simulink model "both_MPC_off_grid"  (R2015b)
settings: Solver=ode5  StartTime=0.0  StopTime=5  RelTol=1e-3
libraries: powerlib x27, powerlib_meascontrol x6, powerlib_extras x1
settings Model: Creator=fujitsu  LastModifiedBy=fujitsu

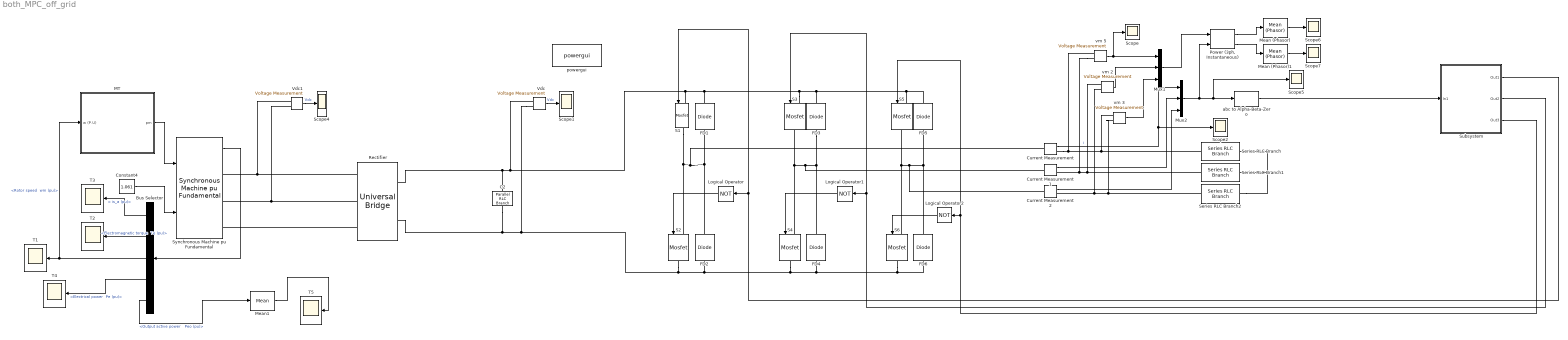
== system both_MPC_off_grid ==
  Bus Selector : BusSelector  OutputSignals="Stator current. is_a (pu),Mechanical.Electromagnetic torque  Te (pu),Mechanical.Rotor speed  wm (pu),Mechanical.Electrical power  Pe (pu),Output active power   Peo (pu)"
  C2 : powerlib/Elements/Parallel RLC Branch  LConnTagsString=a  RConnTagsString=__new0  BranchType=C  Resistance=inf  Inductance=inf  SetiL0=off  InitialCurrent=0  Capacitance=5000e-06  Setx0=off  InitialVoltage=0  Measurements=None
  Constant4 : Constant  Value=1.061
  Current Measurement : powerlib/Measurements/Current Measurement  PhasorSimulation=off  OutputType=Complex  PSBequivalent=0
  Current Measurement1 : powerlib/Measurements/Current Measurement  PhasorSimulation=off  OutputType=Complex  PSBequivalent=0
  Current Measurement2 : powerlib/Measurements/Current Measurement  PhasorSimulation=off  OutputType=Complex  PSBequivalent=0
  FD{1..6} (6 alike) : powerlib/Power Electronics/Diode  Ron=0.001  Lon=0  Vf=0.8  IC=0  UseSnubber=off  Rs=500  Cs=250e-9  Measurements=off
  Logical Operator : Logic  Operator=NOT  AllPortsSameDT=off  OutDataTypeStr=boolean
  Logical Operator1 : Logic  Operator=NOT  AllPortsSameDT=off  OutDataTypeStr=boolean
  Logical Operator2 : Logic  Operator=NOT  AllPortsSameDT=off  OutDataTypeStr=boolean
  MT : Subsystem
  Mean (Phasor) : powerlib_meascontrol/Measurements/Mean (Phasor)  Freq=50  Vinit=0  Ts=0
  Mean (Phasor)1 : powerlib_meascontrol/Measurements/Mean (Phasor)  Freq=50  Vinit=0  Ts=0
  Mean1 : powerlib_meascontrol/Measurements/Mean  Freq=50  Vinit=0  Ts=1e-6
  Mux1 : Mux  Inputs=3
  Mux2 : Mux  Inputs=3
  "Power (3ph, Instantaneous)" : powerlib_meascontrol/Measurements/Power (3ph, Instantaneous)
  Rectifier : powerlib/Power Electronics/Universal Bridge  Arms=3  SnubberResistance=50  SnubberCapacitance=0.1e-6  Device=Diodes  Ron=1e-3  Lon=0  ForwardVoltages="[  0.8  0.8  ]"  ForwardVoltage=.7  GTOparameters=[ 10e-6 , 20e-6 ]  IGBTparameters=[ 1e-6 , 2e-6 ]  Measurements=Device currents  Measurements_2=None  converterType=Rectifier
  S{1..6} (6 alike) : powerlib/Power Electronics/Mosfet  Ron=0.1  Lon=0  Rd=0.01  Vfd=0  IC=0  Rs=1e5  Cs=inf  Measurements=off
  Scope{,1..2,4..7} (7 alike) : Scope
  Series RLC Branch : powerlib/Elements/Series RLC Branch  LConnTagsString=__new0  RConnTagsString=__new0  BranchType=RL  Resistance=765^2/50000  Inductance=10e-3  SetiL0=off  InitialCurrent=0  Capacitance=1e-6  Setx0=off  InitialVoltage=0  Measurements=None
  Series RLC Branch1 : powerlib/Elements/Series RLC Branch  LConnTagsString=__new0  RConnTagsString=__new0  BranchType=RL  Resistance=765^2/50000  Inductance=10e-3  SetiL0=off  InitialCurrent=0  Capacitance=1e-6  Setx0=off  InitialVoltage=0  Measurements=None
  Series RLC Branch2 : powerlib/Elements/Series RLC Branch  LConnTagsString=__new0  RConnTagsString=__new0  BranchType=RL  Resistance=765^2/50000  Inductance=10e-3  SetiL0=off  InitialCurrent=0  Capacitance=1e-6  Setx0=off  InitialVoltage=0  Measurements=None
  Subsystem : Subsystem
  Synchronous Machine pu Fundamental : powerlib/Machines/Synchronous Machine pu Fundamental  PresetModel=No  MechanicalLoad=Mechanical power Pm  ShowDetailedParameters=on  RotorType=Salient-pole  Units=per unit fundamental parameters  MeasurementBus=off  NominalParameters="[ 65e3  580 1600]"  Stator="[ 0.2503  0.114  0.6875  0.6875 ]"  Field="[ 1  10e15/(100*pi)]"  Dampers2=[0.0652, 0.5134, 0.0287, 0.2553, 7.765e-3, 0.9167 ]  Dampers1="[ 1.17E-02  0.182  1.97E-02  0.384 ]"  Mechanical=[ 6 0 2]  PolePairs=20  InitialConditions="[ 0  0  0  0  0  0  0  0  1 ]"  SetSaturation=off  Saturation=[0.6404,0.7127,0.8441,0.9214,0.9956,1.082,1.19,1.316,1.457;0.7,0.7698,0.8872,0.9466,0.9969,1.046,1.1,1.151,1.201]  LoadFlowParameters=[1,0,0,0,0]  TsPowergui=0  TsBlock=-1  IterativeModel=Trapezoidal non iterative  BusType=swing  Pref=0  Qref=0  Qmin=-inf  Qmax=inf  PLF=0  QLF=0
  T{1..5} (5 alike) : Scope
  Vdc : powerlib/Measurements/Voltage Measurement  Tag=PoWeRsYsTeMmEaSuReMeNt  PhasorSimulation=off  OutputType=Magnitude  PSBequivalent=0
  Vdc1 : powerlib/Measurements/Voltage Measurement  Tag=PoWeRsYsTeMmEaSuReMeNt  PhasorSimulation=off  OutputType=Magnitude  PSBequivalent=0
  abc to Alpha-Beta-Zero : powerlib_meascontrol/Transformations/abc to Alpha-Beta-Zero
  powergui : powerlib/powergui  SimulationMode=Continuous  SolverType=Tustin  SampleTime=5e-6  frequency=60  SPID=off  DisableSnubberDevices=off  DisableRonSwitches=off  DisableVfSwitches=off  SwTol=0  DisplayEquations=off  Interpol=off  ExternalGateDelay=off  methode=off  Ts=0  FunctionMessages=off  echomessages=off  HookPort=off  EnableUseOfTLC=off  x0status=blocks  frequencyindice=0  Pbase=100e6  ErrMax=0.0001  Iterations=50  UnitsV=kV  UnitsW=MW  buscounter=0  RestoreLinks=warning  ResistiveCurrentMeasurement=off  Frange=[0:2:500]  Ylog=off  Xlog=on  ShowGrid=off  save=off  variable=ZData  structure=ScopeData11111  ZoomFFT=off  StartTime=2  cycles=5  DisplayStyle=1  fundamental=50  FreqAxis=on  MaxFrequency=10000  frequencyindicesteady=1  RmsSteady=1  display=off
  vm 2 : powerlib/Measurements/Voltage Measurement  PhasorSimulation=off  OutputType=Complex  PSBequivalent=0
  vm 3 : powerlib/Measurements/Voltage Measurement  PhasorSimulation=off  OutputType=Complex  PSBequivalent=0
  vm 5 : powerlib/Measurements/Voltage Measurement  PhasorSimulation=off  OutputType=Complex  PSBequivalent=0
  wires:
  Vdc/1 -> Scope1/1  "Vdc"
  MT/1(pm) -> Synchronous Machine pu Fundamental/1
  Synchronous Machine pu Fundamental/1 -> Bus Selector/1
  Bus Selector/1 -> T3/1  "< is_a (pu)>"
  Bus Selector/2 -> T2/1  "<Electromagnetic torque  Te (pu)>"
  Bus Selector/3 -> MT/1(w (P.U)), T1/1  "<Rotor speed  wm (pu)>"
  Constant4/1 -> Synchronous Machine pu Fundamental/2
  Vdc1/1 -> Scope4/1  "Vdc"
  Bus Selector/4 -> T4/1  "<Electrical power  Pe (pu)>"
  Bus Selector/5 -> Mean1/1  "<Output active power   Peo (pu)>"
  Mean1/1 -> T5/1
  Current Measurement/1 -> Mux2/1, Scope2/1  "i"
  Current Measurement1/1 -> Mux2/2
  Current Measurement2/1 -> Mux2/3
  Mux2/1 -> "Power (3ph, Instantaneous)"/2, Scope5/1, abc to Alpha-Beta-Zero/1
  Logical Operator/1 -> S2/1
  Logical Operator1/1 -> S4/1
  Logical Operator2/1 -> S6/1
  vm 5/1 -> Scope/1, Mux1/1
  Subsystem/3(Out3) -> S5/1, Logical Operator2/1
  Subsystem/2(Out2) -> S3/1, Logical Operator1/1
  Subsystem/1(Out1) -> S1/1, Logical Operator/1
  abc to Alpha-Beta-Zero/1 -> Subsystem/1(In1)
  vm 2/1 -> Mux1/2
  vm 3/1 -> Mux1/3
  Mux1/1 -> "Power (3ph, Instantaneous)"/1
  "Power (3ph, Instantaneous)"/1 -> Mean (Phasor)/1
  "Power (3ph, Instantaneous)"/2 -> Mean (Phasor)1/1
  Mean (Phasor)/1 -> Scope6/1
  Mean (Phasor)1/1 -> Scope7/1
  connections:
  Current Measurement/RConn1 -- vm 5/LConn1 -- vm 3/LConn1 -- Series RLC Branch/LConn1
  S1/RConn1 -- S2/LConn1 -- Current Measurement/LConn1 -- FD1/LConn1 -- FD2/RConn1
  S3/RConn1 -- S4/LConn1 -- FD4/RConn1 -- FD3/LConn1 -- Current Measurement1/LConn1
  S5/RConn1 -- S6/LConn1 -- FD6/RConn1 -- FD5/LConn1 -- Current Measurement2/LConn1
  vm 5/LConn2 -- Current Measurement1/RConn1 -- Series RLC Branch1/LConn1 -- vm 2/LConn1
  Series RLC Branch1/RConn1 -- Series RLC Branch/RConn1 -- Series RLC Branch2/RConn1
  vm 2/LConn2 -- Current Measurement2/RConn1 -- Series RLC Branch2/LConn1 -- vm 3/LConn2
  Synchronous Machine pu Fundamental/RConn1 -- Vdc1/LConn1 -- Rectifier/LConn1
  Vdc/LConn2 -- Rectifier/RConn2 -- C2/RConn1 -- S2/RConn1 -- FD2/LConn1 -- S4/RConn1 -- S6/RConn1 -- FD6/LConn1 -- FD4/LConn1
  S3/LConn1 -- FD1/RConn1 -- Rectifier/RConn1 -- C2/LConn1 -- Vdc/LConn1 -- S1/LConn1 -- FD3/RConn1 -- FD5/RConn1 -- S5/LConn1
  Rectifier/LConn2 -- Vdc1/LConn2 -- Synchronous Machine pu Fundamental/RConn2
  Rectifier/LConn3 -- Synchronous Machine pu Fundamental/RConn3

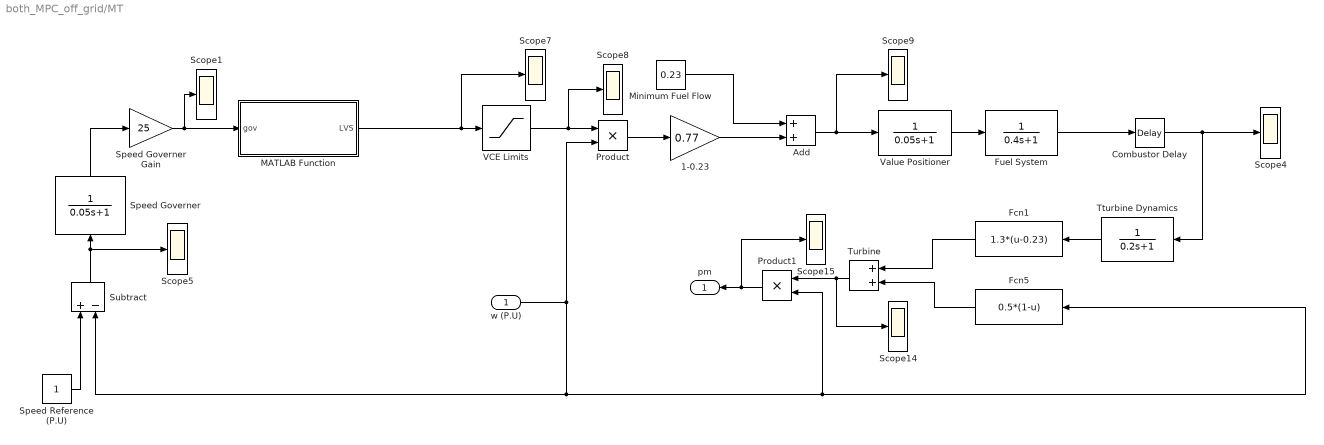
== system both_MPC_off_grid/MT ==
  w (P.U) : Inport
  1-0.23 : Gain  Gain=0.77
  Add : Sum
  Combustor Delay : TransportDelay  DelayTime=0.01
  Fcn1 : Fcn  Expr=1.3*(u-0.23)
  Fcn5 : Fcn  Expr=0.5*(1-u)
  Fuel System : TransferFcn  Denominator=[0.4 1]
  MATLAB Function : MATLAB Function  TreatAsAtomicUnit=on
  Minimum Fuel Flow : Constant  Value=0.23
  Product : Product  RndMeth=Zero
  Product1 : Product  RndMeth=Zero
  Scope{1,4..5,7..9,14..15} (8 alike) : Scope
  Speed Governer : TransferFcn  Denominator=[0.05 1]
  Speed Governer Gain : Gain  Gain=25
  Speed Reference (P.U) : Constant
  Subtract : Sum  Inputs=+-
  Tturbine Dynamics : TransferFcn  Denominator=[0.2 1]
  "Turbine " : Sum
  VCE Limits : Saturate  UpperLimit=1.5  LowerLimit=-0.1
  Value Positioner : TransferFcn  Denominator=[0.05 1]
  pm : Outport
  wires:
  Speed Reference (P.U)/1 -> Subtract/1
  Subtract/1 -> Scope5/1, Speed Governer/1
  VCE Limits/1 -> Scope8/1, Product/1
  Product/1 -> 1-0.23/1
  1-0.23/1 -> Add/2
  Minimum Fuel Flow/1 -> Add/1
  Add/1 -> Scope9/1, Value Positioner/1
  Value Positioner/1 -> Fuel System/1
  Fuel System/1 -> Combustor Delay/1
  Combustor Delay/1 -> Scope4/1, Tturbine Dynamics/1
  Speed Governer Gain/1 -> Scope1/1, MATLAB Function/1(gov)
  Speed Governer/1 -> Speed Governer Gain/1
  w (P.U)/1 -> Product/2, Subtract/2, Product1/2, Fcn5/1
  Tturbine Dynamics/1 -> Fcn1/1
  Fcn1/1 -> "Turbine "/1
  Fcn5/1 -> "Turbine "/2
  Product1/1 -> Scope15/1, pm/1
  "Turbine "/1 -> Scope14/1, Product1/1
  MATLAB Function/1(LVS) -> Scope7/1, VCE Limits/1

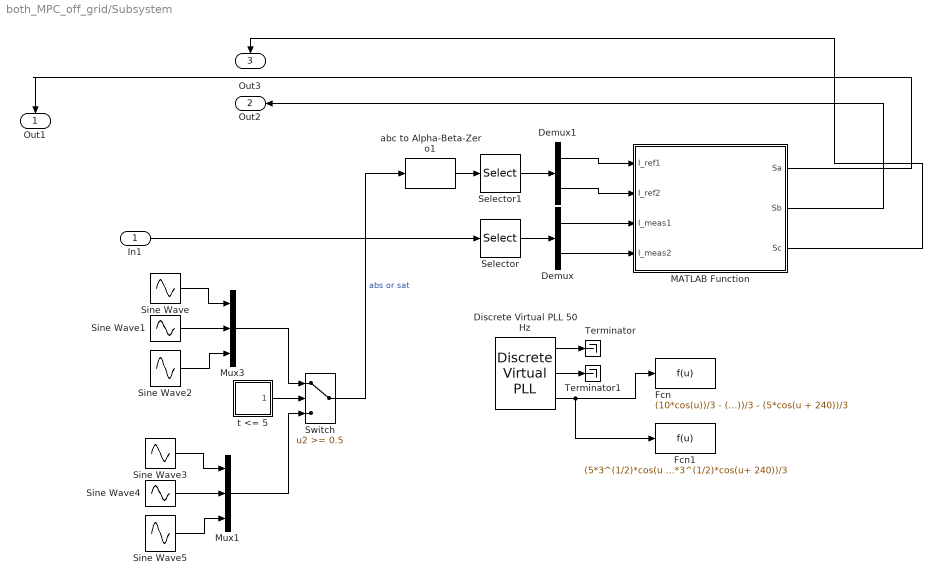
== system both_MPC_off_grid/Subsystem ==
  In1 : Inport
  Demux : Demux  Outputs=2
  Demux1 : Demux  Outputs=2
  Discrete Virtual PLL 50 Hz : powerlib_extras/Discrete  Control Blocks/Discrete Virtual PLL  Freq=50  Phase=0  Ts=30e-6
  Fcn : Fcn  Expr=(10*cos(u))/3 - (5*cos(u + 120))/3 - (5*cos(u + 240))/3
  Fcn1 : Fcn  Expr=(5*3^(1/2)*cos(u + 120))/3 - (5*3^(1/2)*cos(u+ 240))/3
  MATLAB Function : MATLAB Function  TreatAsAtomicUnit=on
  Mux1 : Mux  Inputs=3
  Mux3 : Mux  Inputs=3
  Selector : Selector  InputPortWidth=3  IndexOptions=Index vector (dialog)  Indices=[1 2]  OutputSizes=1
  Selector1 : Selector  InputPortWidth=3  IndexOptions=Index vector (dialog)  Indices=[1 2]  OutputSizes=1
  Sine Wave : Sin  Amplitude=10  Frequency=2*pi*50  SampleTime=0
  Sine Wave1 : Sin  Amplitude=10  Frequency=100*pi  Phase=2*pi/3  SampleTime=0
  Sine Wave2 : Sin  Amplitude=10  Frequency=100*pi  Phase=-2*pi/3  SampleTime=0
  Sine Wave3 : Sin  Amplitude=15  Frequency=2*pi*50  SampleTime=0
  Sine Wave4 : Sin  Amplitude=15  Frequency=100*pi  Phase=2*pi/3  SampleTime=0
  Sine Wave5 : Sin  Amplitude=15  Frequency=100*pi  Phase=-2*pi/3  SampleTime=0
  Switch : Switch  Threshold=0.5  SaturateOnIntegerOverflow=on  InputSameDT=on
  Terminator : Terminator
  Terminator1 : Terminator
  abc to Alpha-Beta-Zero1 : powerlib_meascontrol/Transformations/abc to Alpha-Beta-Zero
  t <= 5 : Subsystem
  Out1 : Outport
  Out2 : Outport  Port=2
  Out3 : Outport  Port=3
  wires:
  In1/1 -> Selector/1
  Selector/1 -> Demux/1
  Demux/1 -> MATLAB Function/3(I_meas1)
  Demux/2 -> MATLAB Function/4(I_meas2)
  MATLAB Function/1(Sa) -> Out1/1
  MATLAB Function/2(Sb) -> Out2/1
  MATLAB Function/3(Sc) -> Out3/1
  Discrete Virtual PLL 50 Hz/1 -> Terminator/1
  Discrete Virtual PLL 50 Hz/2 -> Terminator1/1
  Discrete Virtual PLL 50 Hz/3 -> Fcn1/1, Fcn/1
  abc to Alpha-Beta-Zero1/1 -> Selector1/1
  Selector1/1 -> Demux1/1
  Demux1/1 -> MATLAB Function/1(I_ref1)
  Demux1/2 -> MATLAB Function/2(I_ref2)
  t <= 5/1(t <= 1) -> Switch/2
  Sine Wave/1 -> Mux3/1
  Sine Wave1/1 -> Mux3/2
  Sine Wave2/1 -> Mux3/3
  Sine Wave3/1 -> Mux1/1
  Sine Wave4/1 -> Mux1/2
  Sine Wave5/1 -> Mux1/3
  Mux3/1 -> Switch/1
  Mux1/1 -> Switch/3
  Switch/1 -> abc to Alpha-Beta-Zero1/1  "abs or sat"

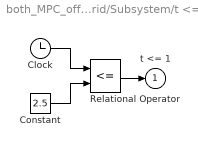
== system both_MPC_off_grid/Subsystem/t <= 5 ==
  Clock : Clock
  Constant : Constant  Value=2.5
  Relational Operator : RelationalOperator  Operator=<=  InputSameDT=on
  t <= 1 : Outport  InitialOutput=0
  wires:
  Constant/1 -> Relational Operator/2
  Clock/1 -> Relational Operator/1
  Relational Operator/1 -> t <= 1/1

== matlab function both_MPC_off_grid/MT/MATLAB Function ==
  data: gov input; LVS output
function LVS= MT(gov)
T=1000e-6;
wref=1;
W=25;
X=0;
Y=0.05;
Z=1;
a1=wref-0.985;
a2=wref-0.986;
a3=wref-0.987;
a4=wref-0.988;
a5=wref-0.989;
a6=wref-0.990;
a7=wref-0.991;
a8=wref-0.992;
a9=wref-0.993;
a10=wref-0.994;
a11=wref-0.995;
a12=wref-0.996;
a13=wref-0.997;
a14=wref-0.998;
a15=wref-0.999;
a16=wref-1;
a17=wref-1.001;
a18=wref-1.002;
a19=wref-1.003;
a20=wref-1.004;
a21=wref-1.005;
a=[a1 a2 a3 a4 a5 a6 a7 a8 a9 a10 a11 a12 a13 a14 a15 a16 a17 a18 a19 a20 a21];
g=zeros(1,21);
for i=1:21
    A=a(i);
  gov=(W*T*A)/Y+gov*(1-(Z*T)/Y);
  g(i)=gov;
end
[y,x]=min(g);
LVS=y;

== matlab function both_MPC_off_grid/Subsystem/MATLAB Function ==
  data: I_ref1 input; Sa output; I_ref2 input; I_meas1 input; I_meas2 input; Sb output; Sc output
function [Sa,Sb,Sc]=MPC(I_ref1,I_ref2,I_meas1,I_meas2)
Ts=25e-6;
R=765^2/50000;
L=10e-3;
e=100;
Vdc=500;
v0=0;
v1=2/3*Vdc;
v2=1/3*Vdc+1j*sqrt(3)/3*Vdc;
v3=-1/3*Vdc+1j*sqrt(3)/3*Vdc;
v4=-2/3*Vdc;
v5=-1/3*Vdc-1j*sqrt(3)/3*Vdc;
v6=1/3*Vdc-1j*sqrt(3)/3*Vdc;
v7=0;
v=[v0 v1 v2 v3 v4 v5 v6 v7]; %standars vector
states=[0 0 0;1 0 0;1 1 0;0 1 0;0 1 1;0 0 1;1 0 1;1 1 1]; %based on SVM standard vectors
persistent x_old i_old 
if isempty(x_old), x_old=1; end
if isempty(i_old), i_old=0+1j*0; end
g=zeros(1,8); 
ik_ref=I_ref1+1j*I_ref2;  %I_ref ha moalefe haye alfa va beta hastand
ik=I_meas1+1j*I_meas2;    
e=v(x_old)-L/Ts*ik-(R-L/Ts)*i_old;
i_old=ik;
for i=1:8
v_o1=v(i); 
ik1=(1-R*Ts/L)*ik+Ts/L*(v_o1-e); 
g(i)=abs(real(ik_ref-ik1))+abs(imag(ik_ref-ik1)); 
end
[yy,x_opt]=min(g); 
x_old=x_opt; 
x_opt=x_old;
Sa=states(x_opt,1);
Sb=states(x_opt,2);
Sc=states(x_opt,3);
